simulink model "empty_MyFilter"  (Simulink 6.3)
settings: Solver=FixedStepDiscrete  SolverMode=SingleTasking  StartTime=0.0  StopTime=500*Tsamp  RelTol=1e-3
PreLoadFcn:
  | init
InitFcn:
  | %% DSPBuilder Start
  | alt_dspbuilder_update_model(bdroot)
  | %% DSPBuilder End
values from neighbouring files (symbols this model uses):
  Tsamp = 1    [init.m]
libraries: allblocks_alteradspbuilder2 x4, simulink x1
settings Model: Creator=gnixon  LastModifiedBy=gnixon

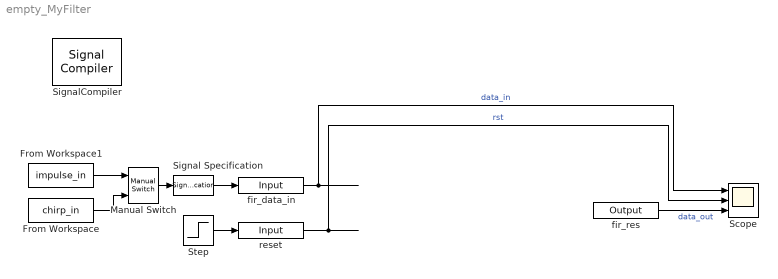
== system empty_MyFilter ==
  From Workspace : FromWorkspace  VariableName=chirp_in  SampleTime=Tsamp
  From Workspace1 : FromWorkspace  VariableName=impulse_in  SampleTime=Tsamp
  Manual Switch : simulink/Signal Routing/Manual Switch  sw=0  action=0
  Scope : Scope  NumInputPorts=3
      settings: YMin=-40000~-1~-1  YMax=40000~1~1
  Signal Specification : SignalSpecification  SampleTime=Tsamp
  SignalCompiler : allblocks_alteradspbuilder2/Signal Compiler  DeviceFamily=Stratix III  DeviceName=AUTO  EnableSignalTap=off  SignalTapDepth=128  UseBoardBlock=off  StpUseDefaultClock=on  StpClock=clock
  Step : Step  Time=3  Before=1  After=0  SampleTime=1
  fir_data_in : allblocks_alteradspbuilder2/Input  iofile=d:\workspaces\dsp_builder\Documentation\DesignExamples\Tutorials\BlackBox\HDLImport\tb_empty_MyFilter\empty_MyFilter_fir_data_in.salt  BusType=Signed Integer  bwl=16  bwr=0  UseDefaultClock=on  PORTTYPE=Input
  fir_res : allblocks_alteradspbuilder2/Output  iofile=d:\workspaces\dsp_builder\Documentation\DesignExamples\Tutorials\BlackBox\HDLImport\tb_empty_MyFilter\empty_MyFilter_fir_res.capture  BusType=Signed Integer  bwl=33  bwr=0  PORTTYPE=Output
  reset : allblocks_alteradspbuilder2/Input  iofile=d:\workspaces\dsp_builder\Documentation\DesignExamples\Tutorials\BlackBox\HDLImport\tb_empty_MyFilter\empty_MyFilter_reset.salt  BusType=Single Bit  bwl=1  bwr=0  UseDefaultClock=on  PORTTYPE=Input
  wires:
  fir_data_in/1 -> Scope/1  "data_in"
  Signal Specification/1 -> fir_data_in/1
  reset/1 -> Scope/2  "rst"
  ? -> fir_res/1
  Step/1 -> reset/1
  fir_res/1 -> Scope/3  "data_out"
  Manual Switch/1 -> Signal Specification/1
  From Workspace1/1 -> Manual Switch/1
  From Workspace/1 -> Manual Switch/2
